simulink model "AIM_OneAgent"  (R2022b)
settings: Solver=ode4  StartTime=0.0  StopTime=inf  FixedStep=0.01  RelTol=1e-3
libraries: simulink x6, slpidlib x4, sim3dautolib x4, rllib x2, sim3dlib x1
(part 2 of 2)

== matlab function AIM_OneAgent/Car_north/Powertrain/Gearbox1 ==
  data: Rg_old input; Rg_new output; Eg_old input; Te input; We input; Wg input; Eg_new output; Tg output; Wt output
function [Rg_new,Eg_new,Tg,Wt] = fcn(Rg_old,Eg_old,Te,We,Wg)
Rg_new=Rg_old;
Eg_new=Eg_old;
if Rg_old == 0
    Rg_new = 2.8;
end
if Eg_old == 0
    Eg_new = 0.94;
end
We = We*(30/pi);
if We>=2500
    if Rg_old == 2.8
        Rg_new = 1.6;
        Eg_new = 0.94;
    elseif Rg_old == 1.6
        Rg_new = 1.1;
        Eg_new = 1;
    elseif Rg_old == 1.1
        Rg_new = 0.8;
        Eg_new = 0.98;
    end
    
elseif We<=1000
    if Rg_old == 0.8
        Rg_new = 1.1;
        Eg_new = 1;
    elseif Rg_old == 1.1
        Rg_new = 1.6;
        Eg_new = 0.94;
    elseif Rg_old == 1.6
        Rg_new = 2.8;
        Eg_new = 0.94;
    end
end
Wt = Wg * Rg_new;
Tg = Te * Rg_new * Eg_new;
end

== matlab function AIM_OneAgent/Car_east/MATLAB Function ==
  data: u input; Ut output; Ub output
function [Ut,Ub] = fcn(u)

 if(u>-0.05 && u<0)
      Ub=0;
      Ut=0;
 elseif(u<-0.05 && u<0)
 Ut=0;
 Ub=-u;
  else
 Ut=u;
 Ub=0;
%  end
 end

== matlab function AIM_OneAgent/Car_north/Powertrain/engine/engine/MATLAB Function ==
  data: alpha input; Te output; Pmax input; Wo input; We input
function Te = fcn(alpha , Pmax , Wo , We)
if We < 500*(pi/30)
    We = 500*(pi/30);
elseif We > 6000*(pi/30)
    We = 6000*(pi/30);
end
Te = (alpha * Pmax * (Wo^2 + We*Wo - We^2)) / (Wo^3);

end

== matlab function AIM_OneAgent/Car_west/MATLAB Function ==
  data: u input; Ut output; Ub output
function [Ut,Ub] = fcn(u)

 if(u>-0.05 && u<0)
      Ub=0;
      Ut=0;
 elseif(u<-0.05 && u<0)
 Ut=0;
 Ub=-u;
  else
 Ut=u;
 Ub=0;
%  end
 end

== matlab function AIM_OneAgent/Car_west/MATLAB Function1 ==
  data: F_aero input; a output; Rx input; Tt input; T_br input
function a = fcn(F_aero , Rx , Tt , T_br)

m = 1400;
Iw = 1.5;
reff = 0.32;

% a = (Tt - T_br - ( (F_aero + Rx)*reff) ) / (m*reff + Iw/reff);

M = (m*reff)+(Iw/reff);
a = (Tt-T_br-reff*(F_aero+Rx))/M;

end

== matlab function AIM_OneAgent/MATLAB Function ==
  data: observation input; reward output; collided input; isdone output
function [reward,isdone] = reward(observation, collided)

x = observation(2);
v = observation(1);

madeit = 0;
if x <= -184.60
    madeit = 1;
else
    madeit = 0;
end
% calculate reward value
collision_penalty = -4000*collided;
arrival_reward = 1000*madeit;

distance = abs(-184.60 - x);

velocity_penalty = -35 * (1 - v/20); % Penalty increases as velocity decreases
distance_reward = 50 * (1 - distance/164); % Reward increases as distance decreases

flag = observation(9);
stopping_early_penalty = -1000* (flag && v<5);

reward = velocity_penalty + distance_reward + collision_penalty + arrival_reward + stopping_early_penalty;

% done if either failed (crashed) or succeeded
isdone = collided || madeit;

== matlab function AIM_OneAgent/Car_west/Powertrain/Gearbox1 ==
  data: Rg_old input; Rg_new output; Eg_old input; Te input; We input; Wg input; Eg_new output; Tg output; Wt output
function [Rg_new,Eg_new,Tg,Wt] = fcn(Rg_old,Eg_old,Te,We,Wg)
Rg_new=Rg_old;
Eg_new=Eg_old;
if Rg_old == 0
    Rg_new = 2.8;
end
if Eg_old == 0
    Eg_new = 0.94;
end
We = We*(30/pi);
if We>=2500
    if Rg_old == 2.8
        Rg_new = 1.6;
        Eg_new = 0.94;
    elseif Rg_old == 1.6
        Rg_new = 1.1;
        Eg_new = 1;
    elseif Rg_old == 1.1
        Rg_new = 0.8;
        Eg_new = 0.98;
    end
    
elseif We<=1000
    if Rg_old == 0.8
        Rg_new = 1.1;
        Eg_new = 1;
    elseif Rg_old == 1.1
        Rg_new = 1.6;
        Eg_new = 0.94;
    elseif Rg_old == 1.6
        Rg_new = 2.8;
        Eg_new = 0.94;
    end
end
Wt = Wg * Rg_new;
Tg = Te * Rg_new * Eg_new;
end

== matlab function AIM_OneAgent/Car_west/Powertrain/engine/engine/MATLAB Function ==
  data: alpha input; Te output; Pmax input; Wo input; We input
function Te = fcn(alpha , Pmax , Wo , We)
if We < 500*(pi/30)
    We = 500*(pi/30);
elseif We > 6000*(pi/30)
    We = 6000*(pi/30);
end
Te = (alpha * Pmax * (Wo^2 + We*Wo - We^2)) / (Wo^3);

end

== matlab function AIM_OneAgent/Car_south/MATLAB Function3 ==
  data: v_ref output
function v_ref = fcn()

v_ref = randi([0, 25]);
end

== matlab function AIM_OneAgent/MATLAB Function1 ==
  data: observation input; reward output; collided input; isdone output
function [reward,isdone] = reward(observation, collided)

x = observation(2);
v = observation(1);

madeit = 0;
if x <= -184.60
    madeit = 1;
else
    madeit = 0;
end
% calculate reward value
collision_penalty = -4000*collided;
arrival_reward = 1000*madeit;

distance = abs(-184.60 - x);

velocity_penalty = -35 * (1 - v/20); % Penalty increases as velocity decreases
distance_reward = 50 * (1 - distance/164); % Reward increases as distance decreases

reward = velocity_penalty + distance_reward + collision_penalty + arrival_reward;

% done if either failed (crashed) or succeeded
isdone = collided || madeit;

== matlab function AIM_OneAgent/MATLAB Function2 ==
  data: dist_es input; v output; dist_en input; xs input; xn input
function v = fcn(dist_es,dist_en,xs,xn)

if (dist_es >= 40 && dist_en >= 40) || (xs > 3 && xn < -3)
    v = 15;
else
    v= 0;
end
end

== matlab function AIM_OneAgent/Car_south/MATLAB Function ==
  data: u input; Ut output; Ub output
function [Ut,Ub] = fcn(u)

 if(u>-0.05 && u<0)
      Ub=0;
      Ut=0;
 elseif(u<-0.05 && u<0)
 Ut=0;
 Ub=-u;
  else
 Ut=u;
 Ub=0;
%  end
 end

== matlab function AIM_OneAgent/Car_east/Powertrain/Gearbox1 ==
  data: Rg_old input; Rg_new output; Eg_old input; Te input; We input; Wg input; Eg_new output; Tg output; Wt output
function [Rg_new,Eg_new,Tg,Wt] = fcn(Rg_old,Eg_old,Te,We,Wg)
Rg_new=Rg_old;
Eg_new=Eg_old;
if Rg_old == 0
    Rg_new = 2.8;
end
if Eg_old == 0
    Eg_new = 0.94;
end
We = We*(30/pi);
if We>=2500
    if Rg_old == 2.8
        Rg_new = 1.6;
        Eg_new = 0.94;
    elseif Rg_old == 1.6
        Rg_new = 1.1;
        Eg_new = 1;
    elseif Rg_old == 1.1
        Rg_new = 0.8;
        Eg_new = 0.98;
    end
    
elseif We<=1000
    if Rg_old == 0.8
        Rg_new = 1.1;
        Eg_new = 1;
    elseif Rg_old == 1.1
        Rg_new = 1.6;
        Eg_new = 0.94;
    elseif Rg_old == 1.6
        Rg_new = 2.8;
        Eg_new = 0.94;
    end
end
Wt = Wg * Rg_new;
Tg = Te * Rg_new * Eg_new;
end

== matlab function AIM_OneAgent/Car_east/MATLAB Function1 ==
  data: F_aero input; a output; Rx input; Tt input; T_br input
function a = fcn(F_aero , Rx , Tt , T_br)

m = 1400;
Iw = 1.5;
reff = 0.32;

% a = (Tt - T_br - ( (F_aero + Rx)*reff) ) / (m*reff + Iw/reff);

M = (m*reff)+(Iw/reff);
a = (Tt-T_br-reff*(F_aero+Rx))/M;

end

== matlab function AIM_OneAgent/Car_east/Powertrain/engine/engine/MATLAB Function ==
  data: alpha input; Te output; Pmax input; Wo input; We input
function Te = fcn(alpha , Pmax , Wo , We)
if We < 500*(pi/30)
    We = 500*(pi/30);
elseif We > 6000*(pi/30)
    We = 6000*(pi/30);
end
Te = (alpha * Pmax * (Wo^2 + We*Wo - We^2)) / (Wo^3);

end

== matlab function AIM_OneAgent/Car_south/MATLAB Function1 ==
  data: F_aero input; a output; Rx input; Tt input; T_br input
function a = fcn(F_aero , Rx , Tt , T_br)

m = 1400;
Iw = 1.5;
reff = 0.32;

% a = (Tt - T_br - ( (F_aero + Rx)*reff) ) / (m*reff + Iw/reff);

M = (m*reff)+(Iw/reff);
a = (Tt-T_br-reff*(F_aero+Rx))/M;

end

== matlab function AIM_OneAgent/Car_south/Powertrain/Gearbox1 ==
  data: Rg_old input; Rg_new output; Eg_old input; Te input; We input; Wg input; Eg_new output; Tg output; Wt output
function [Rg_new,Eg_new,Tg,Wt] = fcn(Rg_old,Eg_old,Te,We,Wg)
Rg_new=Rg_old;
Eg_new=Eg_old;
if Rg_old == 0
    Rg_new = 2.8;
end
if Eg_old == 0
    Eg_new = 0.94;
end
We = We*(30/pi);
if We>=2500
    if Rg_old == 2.8
        Rg_new = 1.6;
        Eg_new = 0.94;
    elseif Rg_old == 1.6
        Rg_new = 1.1;
        Eg_new = 1;
    elseif Rg_old == 1.1
        Rg_new = 0.8;
        Eg_new = 0.98;
    end
    
elseif We<=1000
    if Rg_old == 0.8
        Rg_new = 1.1;
        Eg_new = 1;
    elseif Rg_old == 1.1
        Rg_new = 1.6;
        Eg_new = 0.94;
    elseif Rg_old == 1.6
        Rg_new = 2.8;
        Eg_new = 0.94;
    end
end
Wt = Wg * Rg_new;
Tg = Te * Rg_new * Eg_new;
end

== matlab function AIM_OneAgent/Car_south/Powertrain/engine/engine/MATLAB Function ==
  data: alpha input; Te output; Pmax input; Wo input; We input
function Te = fcn(alpha , Pmax , Wo , We)
if We < 500*(pi/30)
    We = 500*(pi/30);
elseif We > 6000*(pi/30)
    We = 6000*(pi/30);
end
Te = (alpha * Pmax * (Wo^2 + We*Wo - We^2)) / (Wo^3);

end

== matlab function AIM_OneAgent/Calculate Distance ==
  data: xe input; dist output; ye input; xs input; ys input; collided output
function [dist, collided]= calculate_distance(xe,ye,xs,ys)
collided = 0;
dist = sqrt( power(xs-xe,2)+power(ys-ye,2) );
if dist < 5
    collided = 1;
end
end

== matlab function AIM_OneAgent/Calculate Distance1 ==
  data: xe input; dist_es output; dist_en output; ye input; xs input; ys input; collided output; xn input; yn input
function [dist_es, dist_en, collided]= calculate_distance(xe,ye,xs,ys,xn,yn)
collided = 0;
dist_es = sqrt( power(xs-xe,2)+power(ys-ye,2) );
dist_en = sqrt( power(xn-xe,2)+power(yn-ye,2) );
if dist_es < 5 || dist_en < 5
    collided = 1;
end
end
